simulink subsystem "EKF_prediction"  (R2021a)
settings: Solver=VariableStepAuto  StartTime=0.0  StopTime=10.0  RelTol=1e-3
undefined symbols (not defined in the file): imu1, magnitude, Ts
libraries: dspmtrx3 x5
settings Model: Creator=Laura  LastModifiedBy=Laura

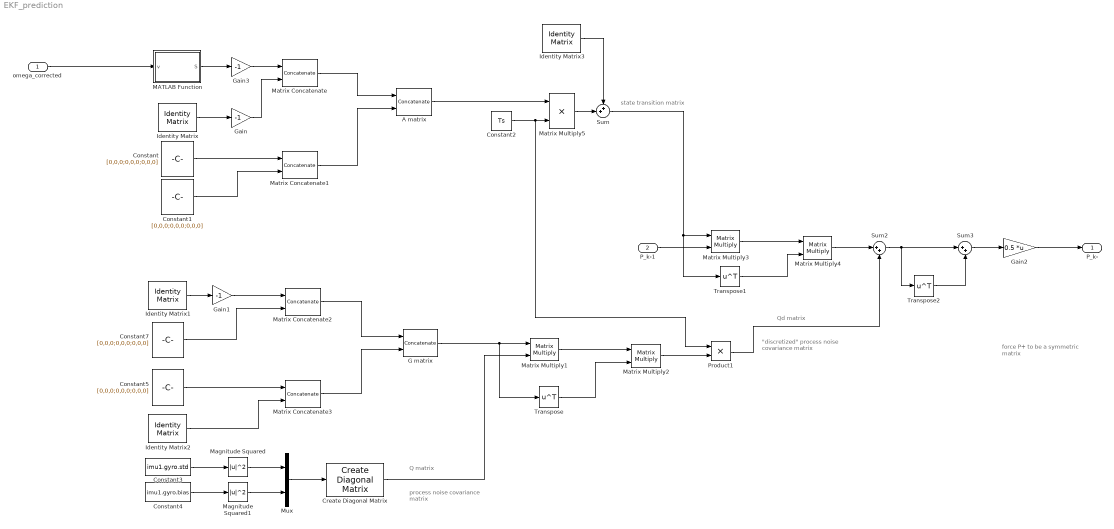
== system EKF_prediction ==
  note: force P+ to be a symmetric matrix
  note: state transition matrix
  note: "discretized" process noise covariance matrix
  note: process noise covariance matrix
  note: Qd matrix
  note: Q matrix
  omega_corrected : Inport
  P_k-1 : Inport  Port=2
  A matrix : Concatenate  Mode=Multidimensional array
  Constant{,1,5,7} (4 alike) : Constant  Value=[0,0,0;0,0,0;0,0,0]
  Constant2 : Constant  Value=Ts
  Constant3 : Constant  Value=imu1.gyro.std
  Constant4 : Constant  Value=imu1.gyro.bias
  Create Diagonal Matrix : dspmtrx3/Create Diagonal Matrix
      settings: SourceProductBaseCode=DS
  G matrix : Concatenate  Mode=Multidimensional array
  Gain : Gain  Gain=-1
  Gain1 : Gain  Gain=-1
  Gain2 : Gain  Gain=0.5  Multiplication=Matrix(K*u)
  Gain3 : Gain  Gain=-1
  Identity Matrix : dspmtrx3/Identity Matrix  Inherit=off  N=3  Ts=1  dataType=double  isSigned=on  wordLen=16  udDataType=sfix(16)  fracBitsMode=Best precision  numFracBits=15  OutDataTypeStr=double  LastOutDataTypeStr=double
  Identity Matrix1 : dspmtrx3/Identity Matrix  Inherit=off  N=3  Ts=1  dataType=double  isSigned=on  wordLen=16  udDataType=sfix(16)  fracBitsMode=Best precision  numFracBits=15  OutDataTypeStr=double  LastOutDataTypeStr=double
  Identity Matrix2 : dspmtrx3/Identity Matrix  Inherit=off  N=3  Ts=1  dataType=double  isSigned=on  wordLen=16  udDataType=sfix(16)  fracBitsMode=Best precision  numFracBits=15  OutDataTypeStr=double  LastOutDataTypeStr=double
  Identity Matrix3 : dspmtrx3/Identity Matrix  Inherit=off  N=6  Ts=1  dataType=double  isSigned=on  wordLen=16  udDataType=sfix(16)  fracBitsMode=Best precision  numFracBits=15  OutDataTypeStr=double  LastOutDataTypeStr=double
  MATLAB Function : MATLAB Function  TreatAsAtomicUnit=on
  Magnitude Squared : Math  Operator=magnitude^2  SaturateOnIntegerOverflow=on
  Magnitude Squared1 : Math  Operator=magnitude^2  SaturateOnIntegerOverflow=on
  Matrix Concatenate{,1..3} (4 alike) : Concatenate  Mode=Multidimensional array  ConcatenateDimension=2
  Matrix Multiply{1..4} (4 alike) : Product  Multiplication=Matrix(*)
  Matrix Multiply5 : Product
  Mux : Mux  Inputs=2
  Product1 : Product
  Sum : Sum  Inputs=++|
  Sum2 : Sum  Inputs=|++
  Sum3 : Sum  Inputs=|++
  Transpose : Math  Operator=transpose  SaturateOnIntegerOverflow=on
  Transpose1 : Math  Operator=transpose  SaturateOnIntegerOverflow=on
  Transpose2 : Math  Operator=transpose  SaturateOnIntegerOverflow=on
  P_k- : Outport
  wires:
  Matrix Multiply5/1 -> Sum/2
  omega_corrected/1 -> MATLAB Function/1(v)
  MATLAB Function/1(S) -> Gain3/1
  Sum/1 -> Transpose1/1, Matrix Multiply3/1
  Gain3/1 -> Matrix Concatenate/1
  Identity Matrix/1 -> Gain/1
  Gain/1 -> Matrix Concatenate/2
  Constant/1 -> Matrix Concatenate1/1
  Constant1/1 -> Matrix Concatenate1/2
  Matrix Concatenate/1 -> A matrix/1
  Matrix Concatenate1/1 -> A matrix/2
  A matrix/1 -> Matrix Multiply5/1
  Constant2/1 -> Matrix Multiply5/2, Product1/1
  Constant5/1 -> Matrix Concatenate3/1
  Identity Matrix1/1 -> Gain1/1
  Gain1/1 -> Matrix Concatenate2/1
  Constant7/1 -> Matrix Concatenate2/2
  Identity Matrix2/1 -> Matrix Concatenate3/2
  Matrix Concatenate2/1 -> G matrix/1
  Matrix Concatenate3/1 -> G matrix/2
  Constant4/1 -> Magnitude Squared1/1
  Magnitude Squared1/1 -> Mux/2
  Magnitude Squared/1 -> Mux/1
  Mux/1 -> Create Diagonal Matrix/1
  Constant3/1 -> Magnitude Squared/1
  G matrix/1 -> Transpose/1, Matrix Multiply1/1
  Create Diagonal Matrix/1 -> Matrix Multiply1/2
  Transpose/1 -> Matrix Multiply2/2
  Matrix Multiply1/1 -> Matrix Multiply2/1
  Matrix Multiply2/1 -> Product1/2
  P_k-1/1 -> Matrix Multiply3/2
  Matrix Multiply3/1 -> Matrix Multiply4/1
  Transpose1/1 -> Matrix Multiply4/2
  Matrix Multiply4/1 -> Sum2/1
  Product1/1 -> Sum2/2
  Sum2/1 -> Transpose2/1, Sum3/1
  Transpose2/1 -> Sum3/2
  Sum3/1 -> Gain2/1
  Gain2/1 -> P_k-/1
  Identity Matrix3/1 -> Sum/1

== matlab function EKF_prediction/MATLAB Function ==
  data: v input; S output
function S = skewm(v)
% skewm forms a skew-symmetric matrix from a 3x1 vector
%
% INPUT
%              v, 3x1 vector
%
%	OUTPUT
%              S, 3x3 skew-symmetric matrix
%
%%
    x = v(1);
    y = v(2);
    z = v(3);

    S = [ 0 -z   y;
          z  0  -x;
         -y  x   0];

end
